simulink model "Physical_Model_Debugger_2"  (R2025b)
settings: Solver=VariableStepAuto  StartTime=0.0  StopTime=100  RelTol=1e-3
values from neighbouring files (symbols this model uses):
  cg_structure = 15 + 5.353e-3    (= 15.005353)    [Final_GA.m]    (also in GA_new_new.m)
  ESC_mass_same = 40e-3    (= 0.04)    [Final_GA.m]    (also in GA_new_new.m)
  g = 9.81    [Final_GA.m]    (also in GA_new_new.m)
  m_counter = 0.15    [Final_GA.m]    (also in GA_new_new.m)
  m_struct = 35.75e-03 * 2    (= 0.0715)    [Final_GA.m]    (also in GA_new_new.m)
  mass_cable = 0.19    [Final_GA.m]    (also in GA_new_new.m)
  miu_k = 0.155    [Final_GA.m]    (also in GA_new_new.m)
  Motor_mass_small = 76e-3    (= 0.076)    [Final_GA.m]    (also in GA_new_new.m)
  prop_mass_small = 6e-3    (= 0.006)    [Final_GA.m]    (also in GA_new_new.m)
undefined symbols (not defined in the file or in its folder): DiscIntNeverNeededParam, m_cart
libraries: simulink x2
settings Model: Creator=adity  LastModifiedBy=adity

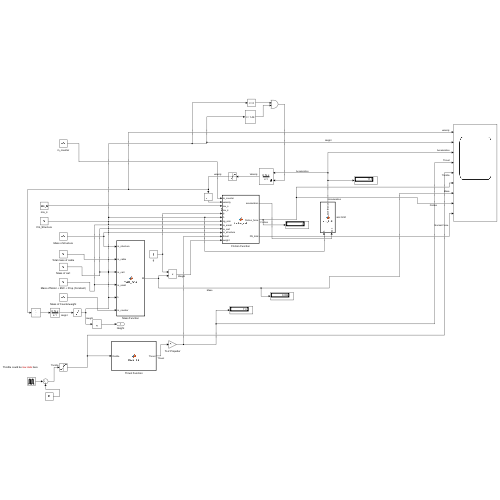
[thumbnail: Simulink's stored preview of the top-level diagram]
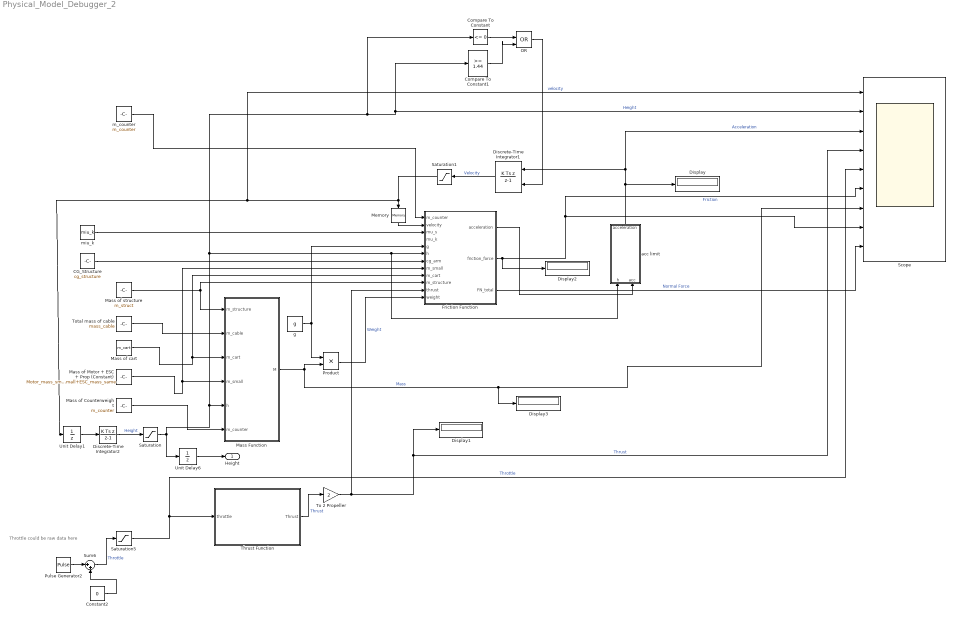
== system Physical_Model_Debugger_2 ==
  note: Throttle could be raw data here
  CG_Structure : Constant  Value=cg_structure
  Compare To Constant : simulink/Logic and Bit Operations/Compare To Constant  relop=<=  const=0  OutDataTypeStr=boolean
  Compare To Constant1 : simulink/Logic and Bit Operations/Compare To Constant  relop=>=  const=1.44  OutDataTypeStr=boolean
  Constant2 : Constant  Value=0
  Discrete-Time Integrator1 : DiscreteIntegrator  IntegratorMethod=Integration: Backward Euler  ExternalReset=rising  SampleTime=0.05  ICPrevOutput=DiscIntNeverNeededParam  ICPrevScaledInput=DiscIntNeverNeededParam
  Discrete-Time Integrator2 : DiscreteIntegrator  IntegratorMethod=Integration: Backward Euler  SampleTime=0.05  ICPrevOutput=DiscIntNeverNeededParam  ICPrevScaledInput=DiscIntNeverNeededParam
  Display{,1..3} (4 alike) : Display
  Friction Function : MATLAB Function  TreatAsAtomicUnit=on
  Mass Function : MATLAB Function  TreatAsAtomicUnit=on
  Mass of Counterweight : Constant  Value=m_counter
  Mass of Motor + ESC + Prop (Constant) : Constant  Value=Motor_mass_small+6*prop_mass_small+ESC_mass_same
  Mass of cart : Constant  Value=m_cart
  Mass of structure : Constant  Value=m_struct
  Memory : Memory
  OR : Logic  Operator=OR  IconShape=distinctive  AllPortsSameDT=off  OutDataTypeStr=boolean
  Product : Product
  Pulse Generator2 : DiscretePulseGenerator  PulseType=Time based  Amplitude=60  Period=10  PulseWidth=5
  Saturation : Saturate  UpperLimit=1.44  LowerLimit=0
  Saturation1 : Saturate  UpperLimit=15  LowerLimit=-15
  Saturation5 : Saturate  UpperLimit=100  LowerLimit=1
  Scope : Scope  NumInputPorts=9
      settings: ActiveDisplayYMinimum=-5.9986461356730416  ActiveDisplayYMaximum=8.7402546513752029
  Sum6 : Sum  Inputs=|++
  Thrust Function : MATLAB Function  TreatAsAtomicUnit=on
  To 2 Propeller : Gain  Gain=2
  Total mass of cable : Constant  Value=mass_cable
  Unit Delay1 : UnitDelay  SampleTime=0.05  HasFrameUpgradeWarning=on
  Unit Delay6 : UnitDelay  SampleTime=0.05  HasFrameUpgradeWarning=on
  acc limit : MATLAB Function  TreatAsAtomicUnit=on
  g : Constant  Value=g
  m_counter : Constant  Value=m_counter
  miu_k : Constant  Value=miu_k
  Height : Outport
  wires:
  Memory/1 -> Friction Function/2(velocity)
  OR/1 -> Discrete-Time Integrator1/2
  Compare To Constant/1 -> OR/1
  Compare To Constant1/1 -> OR/2
  acc limit/1(acceleration) -> Display/1, Discrete-Time Integrator1/1, Scope/3  "Acceleration"
  Saturation5/1 -> Scope/5, Thrust Function/1(throttle)  "Throttle"
  Pulse Generator2/1 -> Sum6/1
  m_counter/1 -> Friction Function/1(m_counter)
  Mass of Motor + ESC + Prop (Constant)/1 -> Mass Function/4(m_small), Friction Function/8(m_small)
  Saturation/1 -> Unit Delay6/1, Compare To Constant/1, Compare To Constant1/1, Scope/2, acc limit/1(h), Friction Function/6(h), Mass Function/5(h)  "Height"
  Constant2/1 -> Sum6/2
  Mass of cart/1 -> Mass Function/3(m_cart), Friction Function/9(m_cart)
  Discrete-Time Integrator2/1 -> Saturation/1  "Height"
  Product/1 -> Friction Function/12(weight)  "Weight"
  Unit Delay6/1 -> Height/1
  g/1 -> Product/1, Friction Function/5(g)
  Total mass of cable/1 -> Mass Function/2(m_cable)
  Mass Function/1(M) -> Product/2, Display3/1, Scope/7  "Mass"
  To 2 Propeller/1 -> Scope/4, Display1/1, Friction Function/11(thrust)  "Thrust"
  Mass of structure/1 -> Mass Function/1(m_structure), Friction Function/10(m_structure)
  Saturation1/1 -> Scope/1, Unit Delay1/1, Memory/1  "velocity"
  Mass of Counterweight/1 -> Mass Function/6(m_counter)
  Thrust Function/1(Thrust) -> To 2 Propeller/1  "Thrust"
  Discrete-Time Integrator1/1 -> Saturation1/1  "Velocity"
  miu_k/1 -> Friction Function/3(mu_s)
  Sum6/1 -> Saturation5/1  "Throttle"
  Unit Delay1/1 -> Discrete-Time Integrator2/1
  CG_Structure/1 -> Friction Function/7(cg_arm)
  Friction Function/1(acceleration) -> acc limit/2(acc)
  Friction Function/2(friction_force) -> Display2/1, Scope/8, Scope/6  "Friction"
  Friction Function/3(FN_total) -> Scope/9  "Normal Force"

== matlab function Physical_Model_Debugger_2/Mass Function ==
  data: m_structure input; m_cable input; m_cart input; m_small input; M output; h input; m_counter input
function M = mass_func(m_structure, m_cable, m_cart, m_small, h, m_counter)
   m_cable_calculated = calculate_cable_mass(h);
    M_cart  = (2 * m_small) + m_cart + m_structure + 2*m_cable_calculated;
    M = M_cart - m_counter;   % effective mass for weight calc
end

function m_supported = calculate_cable_mass(h)

    % --- Physical Constants ---
    m_total = 0.190;        % Total mass of the cable (kg)
    L_total = 1.0;          % Total length of the cable (m)
    y_anchor = 0.33;        % Height of the fixed anchor point (m)
    
    % The height of the attachment point on the cart (from previous equations)
    y_cart = h - 1.052; 

    % The vertical distance between the moving cart and the fixed anchor
    delta_y = y_cart - y_anchor;

    % --- Drag Chain Piecewise Logic ---
    
    if delta_y >= L_total
        % 1. Fully Taut Upward
        % The cart is so high that the entire 1m cable is pulled straight up.
        % The cart supports the entire weight of the cable.
        m_supported = m_total;
        
    elseif delta_y <= -L_total
        % 2. Fully Taut Downward
        % The cart has dropped so low that the cable is pulled straight down.
        % The fixed anchor supports all the weight. (Included for robust simulation bounds).
        m_supported = 0;
        
    else
        % 3. U-Shape / Active Drag Chain Regime
        % The cable forms a U-shape loop. The mass supported by the cart scales 
        % linearly based on the relative height difference.
        
        % Calculate the length of the chain on the cart's side of the "U"
        L_supported = (delta_y + L_total) / 2;
        
        % Convert supported length to supported mass
        m_supported = (m_total / L_total) * L_supported;
    end
end

== matlab function Physical_Model_Debugger_2/Friction Function ==
  data: m_counter input; velocity input; mu_s input; mu_k input; g input; h input; cg_arm input; m_small input; m_cart input; m_structure input; thrust input; weight input; acceleration output; friction_force output; FN_total output
function [acceleration, friction_force, FN_total] = friction_cal( ...
    m_counter, velocity, mu_s, mu_k, g, h, ...
    cg_arm, m_small, m_cart, ...
    m_structure, thrust, weight)

% ============================================================
% Smooth Friction Model for Rail-Mounted Duocopter Cart
%
% Features:
% - Continuous friction law
% - Stribeck transition
% - No hard switching
% - Solver-friendly
% - Includes optional viscous damping
% ============================================================

%% -------------------------
% Geometry / Constants
%% -------------------------

m_cable = 0.095 * h + 0.053656;

y_pad = 0.171;

cg_cart = (7.889 + 27) * 1e-3;

% Small stabilizing preload
FN_bias = 1.27;

% Velocity smoothing parameter
v_s = 0.01;

% Optional viscous damping
c_viscous = 0.2;

%% -------------------------
% Total Inertial Mass
%% -------------------------

m_total = ...
    m_structure + ...
    2*m_small + ...
    m_cart + ...
    m_cable + ...
    m_counter;

%% -------------------------
% External Driving Force
%% -------------------------

F_external = thrust - weight;

%% -------------------------
% Normal Force Calculation
%% -------------------------

% Main cart normal force
FN_cart = abs( ...
    2 * ( ...
        thrust * cg_arm ...
        - (m_structure + 2*m_small) * g * cg_arm ...
        - (m_cart + m_cable) * g * cg_cart ...
    ) / y_pad ...
);

% Counterweight normal force
FN_counter = abs( ...
    (2 * m_counter * g * cg_cart) / y_pad ...
);

% Total normal force
FN_total = FN_cart + FN_counter + FN_bias;

%% -------------------------
% Friction Limits
%% -------------------------

F_static  = mu_s * FN_total;
F_coulomb = mu_k * FN_total;

%% -------------------------
% Stribeck Friction Model
%% -------------------------

% Smooth transition static -> kinetic
F_stribeck = ...
    F_coulomb + ...
    (F_static - F_coulomb) * exp(-(abs(velocity)/v_s)^2);

% Smooth sign function
smooth_sign = tanh(velocity / v_s);

% Total friction force
friction_force = ...
    -F_stribeck * smooth_sign ...
    - c_viscous * velocity;

%% -------------------------
% Acceleration
%% -------------------------

acceleration = ...
    (F_external + friction_force) / m_total;

end

== matlab function Physical_Model_Debugger_2/Thrust Function ==
  data: throttle input; Thrust output
function Thrust = thrust_cal(throttle)

if throttle >= 0 && throttle <= 79.0425

    Thrust = ...
        -1.02178722e-11 * throttle^7 + ...
         3.31547781e-09 * throttle^6 + ...
        -4.23315827e-07 * throttle^5 + ...
         2.75535168e-05 * throttle^4 + ...
        -9.84949443e-04 * throttle^3 + ...
         1.84147041e-02 * throttle^2 + ...
        -2.92219275e-02 * throttle + ...
         5.09621010e-02;

elseif throttle > 79.0425 && throttle <= 100

    Thrust = 7.4300463179;

else

    error('Invalid throttle input');

end

end

== matlab function Physical_Model_Debugger_2/acc limit ==
  data: h input; acc input; acceleration output
function acceleration = acc_limit(h,acc)
if h<=0 
    acceleration = max(acc,0);
elseif h>= 1.44
    acceleration = min(acc,0);
else
    acceleration = acc;
end
